simulink model "sim_model"  (R2015b)
settings: Solver=VariableStepAuto  SolverMode=SingleTasking  StartTime=0.0  StopTime=10.0  MaxStep=0.0001  RelTol=1e-3
undefined symbols (not defined in the file): A_et, A_ou, A_r, B_et, B_ou, B_r
settings Model: Creator=yktma  LastModifiedBy=bedla
settings DataIOCC: ExternalInput=signal  LimitDataPoints=off  LoadExternalInput=on  ReturnWorkspaceOutputs=on
settings DebuggingCC: AllowSymbolicDim=on  SFUnexpectedBacktrackingDiag=error  SFNoUnconditionalDefaultTransitionDiag=error
settings ModelReferenceCC: PropagateSignalLabelsOutOfModel=on
settings SFSimCC: SimUseLocalCustomCode=on
settings RTWCC: RTWUseLocalCustomCode=on
settings GRTTargetCC: TargetLangStandard=C99 (ISO)
settings ConfigComp: CovMetricSettings=dwe  CovHtmlReporting=off  CovSaveCumulativeToWorkspaceVar=off  CovSaveSingleToWorkspaceVar=off  CovModelRefEnable=Off  CovExternalEMLEnable=on

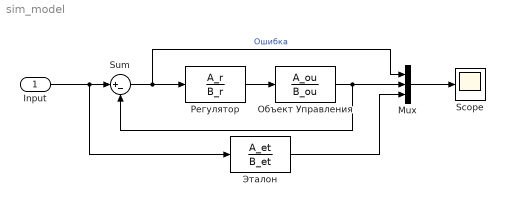
== system sim_model ==
  Input : Inport
  Mux : Mux  Inputs=3
  Scope : Scope
  Sum : Sum  Inputs=|+-
  Объект Управления : TransferFcn  Numerator=A_ou  Denominator=B_ou
  Регулятор : TransferFcn  Numerator=A_r  Denominator=B_r
  Эталон : TransferFcn  Numerator=A_et  Denominator=B_et
  wires:
  Input/1 -> Эталон/1, Sum/1
  Sum/1 -> Mux/1, Регулятор/1  "Ошибка"
  Регулятор/1 -> Объект Управления/1
  Эталон/1 -> Mux/3
  Объект Управления/1 -> Sum/2, Mux/2
  Mux/1 -> Scope/1
